simulink model "Week2"  (R2016b)
settings: Solver=FixedStepDiscrete  StartTime=0.0  StopTime=inf  FixedStep=0.5  RelTol=1e-3  EnableMultiTasking=on
model workspace (MAT data in the model file):
  Backward = -1
  False = 0
  Forward = 1
  Green = 1
  Red = 0
  Stop = 0
  True = 1
settings Model: Creator=troy  LastModifiedBy=troy
settings SolverCC: AutoInsertRateTranBlk=on
settings DataIOCC: LimitDataPoints=on
settings OptimizationCC: LifeSpan=inf
settings DebuggingCC: AllowSymbolicDim=off  SFUnexpectedBacktrackingDiag=warning  SFNoUnconditionalDefaultTransitionDiag=warning  SFExecutionAtInitializationDiag=none
settings GRTTargetCC: TargetLangStandard=C89/C90 (ANSI)  GeneratePreprocessorConditionals=Disable all
settings ConfigComp: CovMetricSettings=dw  CovHtmlReporting=on  CovSaveCumulativeToWorkspaceVar=on  CovSaveSingleToWorkspaceVar=on  CovExternalEMLEnable=off  CovSFcnEnable=off

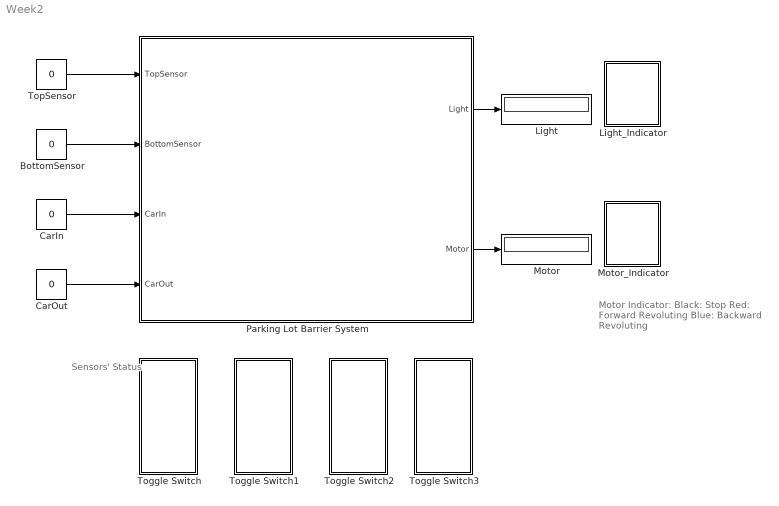
== system Week2 ==
  note: Sensors'
      | Status
  note: Motor Indicator:
      | Black: Stop
      | Red: Forward Revoluting
      | Blue: Backward Revoluting
  BottomSensor : Constant  Value=0
  CarIn : Constant  Value=0
  CarOut : Constant  Value=0
  Light : Display
  Light_Indicator : Subsystem  DialogController=hmiCreateDDGDialog  IsWebBlock=on  mask(MWDashboardBlock){webBlockId=a3b4e4e3-481d-4937-8c1a-36013b46d125, webBlockType=lamp, ShowInLibBrowser=on, ShowInitialText=on, HMISrcModelName=Week2}
      mask prompts: webBlockType "WebBlock Type"; HMISrcModelName "Source Model"
      mask help: SimulinkHMI:dialogs:LampDialogDesc
      mask Help: helpview([docroot '/mapfiles/simulink.map'], 'hmi_lamp')
      mask Display:
      | if strcmp(get_param(bdroot(gcb),'BlockDiagramType'), 'library')
      |     image([(matlabroot) '/toolbox/simulink/hmi/icons/Lamp.png']);
      | end
  Motor : Display
  Motor_Indicator : Subsystem  DialogController=hmiCreateDDGDialog  IsWebBlock=on  mask(MWDashboardBlock){webBlockId=6aca1e5c-966f-43b6-9f83-4e515565c480, webBlockType=lamp, ShowInLibBrowser=on, ShowInitialText=on, HMISrcModelName=Week2}
      mask prompts: webBlockType "WebBlock Type"; HMISrcModelName "Source Model"
      mask help: SimulinkHMI:dialogs:LampDialogDesc
      mask Help: helpview([docroot '/mapfiles/simulink.map'], 'hmi_lamp')
      mask Display:
      | if strcmp(get_param(bdroot(gcb),'BlockDiagramType'), 'library')
      |     image([(matlabroot) '/toolbox/simulink/hmi/icons/Lamp.png']);
      | end
  Parking Lot Barrier System : Stateflow chart  TreatAsAtomicUnit=on
  Toggle Switch : Subsystem  DialogController=hmiCreateDDGDialog  IsWebBlock=on  mask(MWDashboardBlock){webBlockId=e655cf1f-384d-494f-bc9f-979341c9e4ea, webBlockType=toggleswitch, ShowInLibBrowser=on, ShowInitialText=on, HMISrcModelName=Week2}
      mask prompts: webBlockId "WebBlock Id"; webBlockType "WebBlock Type"; HMISrcModelName "Source Model"
      mask help: SimulinkHMI:dialogs:SwitchDialogDesc
      mask Help: helpview([docroot '/mapfiles/simulink.map'], 'hmi_toggle_switch')
      mask Display:
      | if strcmp(get_param(bdroot(gcb),'BlockDiagramType'), 'library')
      |     image([(matlabroot) '/toolbox/simulink/hmi/icons/ToggleSwitch.png']);
      | end
  Toggle Switch1 : Subsystem  DialogController=hmiCreateDDGDialog  IsWebBlock=on  mask(MWDashboardBlock){webBlockId=9cff68f4-5553-4c1b-9417-3c8778fc425a, webBlockType=toggleswitch, ShowInLibBrowser=on, ShowInitialText=on, HMISrcModelName=Week2}
      mask prompts: webBlockId "WebBlock Id"; webBlockType "WebBlock Type"; HMISrcModelName "Source Model"
      mask help: SimulinkHMI:dialogs:SwitchDialogDesc
      mask Help: helpview([docroot '/mapfiles/simulink.map'], 'hmi_toggle_switch')
      mask Display:
      | if strcmp(get_param(bdroot(gcb),'BlockDiagramType'), 'library')
      |     image([(matlabroot) '/toolbox/simulink/hmi/icons/ToggleSwitch.png']);
      | end
  Toggle Switch2 : Subsystem  DialogController=hmiCreateDDGDialog  IsWebBlock=on  mask(MWDashboardBlock){webBlockId=3efde161-6e65-4fd9-a628-429ebcac0e68, webBlockType=toggleswitch, ShowInLibBrowser=on, ShowInitialText=on, HMISrcModelName=Week2}
      mask prompts: webBlockId "WebBlock Id"; webBlockType "WebBlock Type"; HMISrcModelName "Source Model"
      mask help: SimulinkHMI:dialogs:SwitchDialogDesc
      mask Help: helpview([docroot '/mapfiles/simulink.map'], 'hmi_toggle_switch')
      mask Display:
      | if strcmp(get_param(bdroot(gcb),'BlockDiagramType'), 'library')
      |     image([(matlabroot) '/toolbox/simulink/hmi/icons/ToggleSwitch.png']);
      | end
  Toggle Switch3 : Subsystem  DialogController=hmiCreateDDGDialog  IsWebBlock=on  mask(MWDashboardBlock){webBlockId=409f7fc1-c625-4ce2-804b-54fa23253515, webBlockType=toggleswitch, ShowInLibBrowser=on, ShowInitialText=on, HMISrcModelName=Week2}
      mask prompts: webBlockId "WebBlock Id"; webBlockType "WebBlock Type"; HMISrcModelName "Source Model"
      mask help: SimulinkHMI:dialogs:SwitchDialogDesc
      mask Help: helpview([docroot '/mapfiles/simulink.map'], 'hmi_toggle_switch')
      mask Display:
      | if strcmp(get_param(bdroot(gcb),'BlockDiagramType'), 'library')
      |     image([(matlabroot) '/toolbox/simulink/hmi/icons/ToggleSwitch.png']);
      | end
  TopSensor : Constant  Value=0
  wires:
  Parking Lot Barrier System/1(Light) -> Light/1
  Parking Lot Barrier System/2(Motor) -> Motor/1
  TopSensor/1 -> Parking Lot Barrier System/1(TopSensor)
  BottomSensor/1 -> Parking Lot Barrier System/2(BottomSensor)
  CarIn/1 -> Parking Lot Barrier System/3(CarIn)
  CarOut/1 -> Parking Lot Barrier System/4(CarOut)

== system Week2/Light_Indicator ==

== system Week2/Motor_Indicator ==

== system Week2/Toggle Switch ==

== system Week2/Toggle Switch1 ==

== system Week2/Toggle Switch2 ==

== system Week2/Toggle Switch3 ==

== stateflow chart Week2/Parking Lot Barrier System ==
  state IdleState
    entry:
    Light = Red
    Motor = Stop
  state BarrierFalling
    entry:
    Motor = Backward
  state BarrierRising
    entry:
    Motor = Forward
  state CarDrving
    entry:
    Light = Green
    Motor = Stop
  (default) -> IdleState
  BarrierFalling -> IdleState : [BottomSensor == True]
  IdleState -> BarrierRising : [CarIn == True]
  BarrierRising -> CarDrving : [TopSensor == True]
  CarDrving -> BarrierFalling : [CarOut == True]
  data: TopSensor input; BottomSensor input; CarIn input; CarOut input; Light output; Motor output; Red parameter; Stop parameter; Backward parameter; Forward parameter; Green parameter; True parameter
